simulink model "mod7b"  (R2021b)
settings: Solver=VariableStepAuto  StartTime=0.0  StopTime=10.0  RelTol=1e-3
values from neighbouring files (symbols this model uses):
  a = 6    [run_mod7b.m]    (also in run_mod7c.m)
  b = -6    [run_mod7b.m]    (also in run_mod7c.m = 6)
  c = -11    [run_mod7b.m]    (also in run_mod7c.m = 11)
  d = -6    [run_mod7b.m]    (also in run_mod7c.m = 6)
settings Model: Creator=anacl  LastModifiedBy=anacl
settings DataIOCC: SaveFormat=Array  ReturnWorkspaceOutputs=off

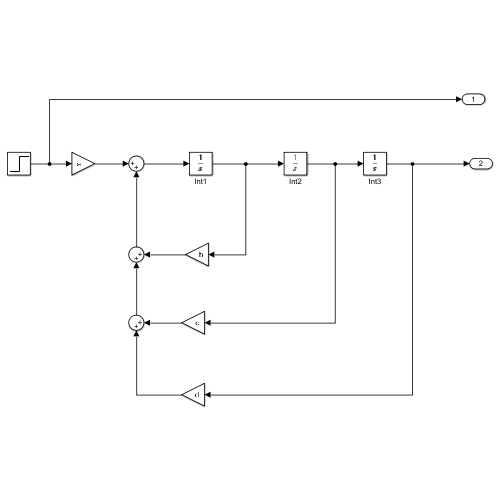
[thumbnail: Simulink's stored preview of the top-level diagram]
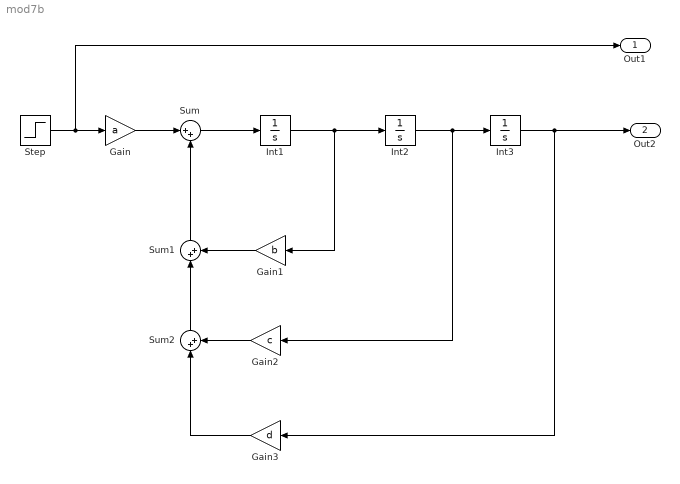
== system mod7b ==
  Gain : Gain  Gain=a
  Gain1 : Gain  Gain=b
  Gain2 : Gain  Gain=c
  Gain3 : Gain  Gain=d
  Int1 : Integrator
  Int2 : Integrator
  Int3 : Integrator  InitialCondition=1
  Step : Step  SampleTime=0
  Sum : Sum  Inputs=|++
  Sum1 : Sum  Inputs=|++
  Sum2 : Sum  Inputs=|++
  Out1 : Outport
  Out2 : Outport  Port=2
  wires:
  Step/1 -> Out1/1, Gain/1
  Gain/1 -> Sum/1
  Sum/1 -> Int1/1
  Int1/1 -> Gain1/1, Int2/1
  Int3/1 -> Out2/1, Gain3/1
  Gain1/1 -> Sum1/2
  Sum1/1 -> Sum/2
  Sum2/1 -> Sum1/1
  Gain3/1 -> Sum2/1
  Gain2/1 -> Sum2/2
  Int2/1 -> Gain2/1, Int3/1
